simulink model "robosimulador"  (R2021b)
settings: Solver=VariableStepAuto  StartTime=0.0  StopTime=Time(length(Time))  MaxStep=1e-3  RelTol=1e-3
model workspace: external: MATLAB File /home/fabio/Desktop/Larc 2021/robosimulador_DataFile.m (data not in the file)
values from neighbouring files (symbols this model uses):
  j = length(Q)    [Cinematica_Comb.m]    (also in Cinematica_Heli_Coronal.m; Cinematica_Heli_Direta_Coronal.m; Cinematica_Heli_Sagital.m)
  Q = Qr    [Cinematica_Comb.m]
  X = zeros(1,14)    [Cinematica_Comb.m]    (also in Cinematica_Heli_Coronal.m = zeros(1,6); Cinematica_Heli_Direta_Coronal.m = zeros(1,6); Cinematica_Heli_Sagital.m = zeros(1,8))
  Y = zeros(1,14)    [Cinematica_Comb.m]    (also in Cinematica_Heli_Coronal.m = zeros(1,6); Cinematica_Heli_Direta_Coronal.m = zeros(1,6); Cinematica_Heli_Sagital.m = zeros(1,8))
  Z = zeros(1,14)    [Cinematica_Comb.m]    (also in Cinematica_Heli_Coronal.m = zeros(1,6); Cinematica_Heli_Direta_Coronal.m = zeros(1,6); Cinematica_Heli_Sagital.m = zeros(1,8))
undefined symbols (not defined in the file or in its folder): g, height_plane, plane_x, smiData, Time, Tmax, zzmp
libraries: nesl_utility x168, sm_lib x117, simulink x38, sharedutil x19, Contact_Forces_Lib x8
(part 6 of 6)

== system robosimulador/Robô/Lado Direito/Centro de Massa/ZMP Quadril/IW bat ==
  Constant1 : Constant  Value=smiData.Solid(10).PoI
  Constant4 : Constant  Value=smiData.Solid(10).MoI
  Demux1 : Demux  Outputs=3
  Demux2 : Demux  Outputs=3
  Gain : Gain  Gain=10e-6
  MATLAB Function1 : MATLAB Function  TreatAsAtomicUnit=on
  Multiply : Product  Multiplication=Matrix(*)
  PS-Simulink Converter1 : nesl_utility/PS-Simulink Converter  PhysicalDomain=network_engine_domain  SubClassName=ps_output  LeftPortType=input  RightPortType=output  PseudoPeriodic=off  Frequencies=[]  Unit=rad  AffineConversion=off
      settings: SourceProductBaseCode=PW,SS
  PS-Simulink Converter7 : nesl_utility/PS-Simulink Converter  PhysicalDomain=network_engine_domain  SubClassName=ps_output  LeftPortType=input  RightPortType=output  PseudoPeriodic=off  Frequencies=[]  Unit=rad/s  AffineConversion=off
      settings: SourceProductBaseCode=PW,SS
  PS-Simulink Converter8 : nesl_utility/PS-Simulink Converter  PhysicalDomain=network_engine_domain  SubClassName=ps_output  LeftPortType=input  RightPortType=output  PseudoPeriodic=off  Frequencies=[]  Unit=rad/s  AffineConversion=off
      settings: SourceProductBaseCode=PW,SS
  PS-Simulink Converter9 : nesl_utility/PS-Simulink Converter  PhysicalDomain=network_engine_domain  SubClassName=ps_output  LeftPortType=input  RightPortType=output  PseudoPeriodic=off  Frequencies=[]  Unit=rad/s  AffineConversion=off
      settings: SourceProductBaseCode=PW,SS
  Vector Concatenate : Concatenate  NumInputs=3
  wx : PMIOPort  Side=Left
  wy : PMIOPort  Port=2  Side=Left
  wz : PMIOPort  Port=3  Side=Left
  R : PMIOPort  Port=4  Side=Left
  Iw : Outport  VectorParamsAs1DForOutWhenUnconnected=off
  wires:
  Demux2/1 -> MATLAB Function1/2(Ix)
  Demux2/3 -> MATLAB Function1/4(Iz)
  PS-Simulink Converter7/1 -> Vector Concatenate/1
  Demux1/1 -> MATLAB Function1/5(Px)
  Demux1/2 -> MATLAB Function1/6(Py)
  Constant1/1 -> Demux1/1
  PS-Simulink Converter8/1 -> Vector Concatenate/2
  Vector Concatenate/1 -> Multiply/2
  PS-Simulink Converter9/1 -> Vector Concatenate/3
  MATLAB Function1/1(Ir) -> Gain/1
  Multiply/1 -> Iw/1
  Demux2/2 -> MATLAB Function1/3(Iy)
  Demux1/3 -> MATLAB Function1/7(Pz)
  Gain/1 -> Multiply/1
  Constant4/1 -> Demux2/1
  PS-Simulink Converter1/1 -> MATLAB Function1/1(R)
  connections:
  PS-Simulink Converter9/LConn1 -- wz/RConn1
  wx/RConn1 -- PS-Simulink Converter7/LConn1
  wy/RConn1 -- PS-Simulink Converter8/LConn1
  PS-Simulink Converter1/LConn1 -- R/RConn1

== system robosimulador/Robô/Lado Direito/Centro de Massa/ZMP Quadril1/IW bat ==
  Constant1 : Constant  Value=smiData.Solid(2).PoI
  Constant4 : Constant  Value=smiData.Solid(2).MoI
  Demux1 : Demux  Outputs=3
  Demux2 : Demux  Outputs=3
  Gain : Gain  Gain=10e-6
  MATLAB Function1 : MATLAB Function  TreatAsAtomicUnit=on
  Multiply : Product  Multiplication=Matrix(*)
  PS-Simulink Converter1 : nesl_utility/PS-Simulink Converter  PhysicalDomain=network_engine_domain  SubClassName=ps_output  LeftPortType=input  RightPortType=output  PseudoPeriodic=off  Frequencies=[]  Unit=rad  AffineConversion=off
      settings: SourceProductBaseCode=PW,SS
  PS-Simulink Converter7 : nesl_utility/PS-Simulink Converter  PhysicalDomain=network_engine_domain  SubClassName=ps_output  LeftPortType=input  RightPortType=output  PseudoPeriodic=off  Frequencies=[]  Unit=rad/s  AffineConversion=off
      settings: SourceProductBaseCode=PW,SS
  PS-Simulink Converter8 : nesl_utility/PS-Simulink Converter  PhysicalDomain=network_engine_domain  SubClassName=ps_output  LeftPortType=input  RightPortType=output  PseudoPeriodic=off  Frequencies=[]  Unit=rad/s  AffineConversion=off
      settings: SourceProductBaseCode=PW,SS
  PS-Simulink Converter9 : nesl_utility/PS-Simulink Converter  PhysicalDomain=network_engine_domain  SubClassName=ps_output  LeftPortType=input  RightPortType=output  PseudoPeriodic=off  Frequencies=[]  Unit=rad/s  AffineConversion=off
      settings: SourceProductBaseCode=PW,SS
  Vector Concatenate : Concatenate  NumInputs=3
  wx : PMIOPort  Side=Left
  wy : PMIOPort  Port=2  Side=Left
  wz : PMIOPort  Port=3  Side=Left
  R : PMIOPort  Port=4  Side=Left
  Iw : Outport  VectorParamsAs1DForOutWhenUnconnected=off
  wires:
  PS-Simulink Converter1/1 -> MATLAB Function1/1(R)
  Constant4/1 -> Demux2/1
  Gain/1 -> Multiply/1
  Demux1/3 -> MATLAB Function1/7(Pz)
  Demux2/2 -> MATLAB Function1/3(Iy)
  Multiply/1 -> Iw/1
  MATLAB Function1/1(Ir) -> Gain/1
  PS-Simulink Converter9/1 -> Vector Concatenate/3
  Vector Concatenate/1 -> Multiply/2
  PS-Simulink Converter8/1 -> Vector Concatenate/2
  Constant1/1 -> Demux1/1
  Demux1/2 -> MATLAB Function1/6(Py)
  Demux1/1 -> MATLAB Function1/5(Px)
  PS-Simulink Converter7/1 -> Vector Concatenate/1
  Demux2/3 -> MATLAB Function1/4(Iz)
  Demux2/1 -> MATLAB Function1/2(Ix)
  connections:
  PS-Simulink Converter1/LConn1 -- R/RConn1
  wy/RConn1 -- PS-Simulink Converter8/LConn1
  wx/RConn1 -- PS-Simulink Converter7/LConn1
  PS-Simulink Converter9/LConn1 -- wz/RConn1

== system robosimulador/Robô/Lado Direito/Centro de Massa/ZMP canela/IW bat ==
  Constant1 : Constant  Value=smiData.Solid(6).PoI
  Constant4 : Constant  Value=smiData.Solid(6).MoI
  Demux1 : Demux  Outputs=3
  Demux2 : Demux  Outputs=3
  Gain : Gain  Gain=10e-6
  MATLAB Function1 : MATLAB Function  TreatAsAtomicUnit=on
  Multiply : Product  Multiplication=Matrix(*)
  PS-Simulink Converter1 : nesl_utility/PS-Simulink Converter  PhysicalDomain=network_engine_domain  SubClassName=ps_output  LeftPortType=input  RightPortType=output  PseudoPeriodic=off  Frequencies=[]  Unit=rad  AffineConversion=off
      settings: SourceProductBaseCode=PW,SS
  PS-Simulink Converter7 : nesl_utility/PS-Simulink Converter  PhysicalDomain=network_engine_domain  SubClassName=ps_output  LeftPortType=input  RightPortType=output  PseudoPeriodic=off  Frequencies=[]  Unit=rad/s  AffineConversion=off
      settings: SourceProductBaseCode=PW,SS
  PS-Simulink Converter8 : nesl_utility/PS-Simulink Converter  PhysicalDomain=network_engine_domain  SubClassName=ps_output  LeftPortType=input  RightPortType=output  PseudoPeriodic=off  Frequencies=[]  Unit=rad/s  AffineConversion=off
      settings: SourceProductBaseCode=PW,SS
  PS-Simulink Converter9 : nesl_utility/PS-Simulink Converter  PhysicalDomain=network_engine_domain  SubClassName=ps_output  LeftPortType=input  RightPortType=output  PseudoPeriodic=off  Frequencies=[]  Unit=rad/s  AffineConversion=off
      settings: SourceProductBaseCode=PW,SS
  Vector Concatenate : Concatenate  NumInputs=3
  wx : PMIOPort  Side=Left
  wy : PMIOPort  Port=2  Side=Left
  wz : PMIOPort  Port=3  Side=Left
  R : PMIOPort  Port=4  Side=Left
  Iw : Outport  VectorParamsAs1DForOutWhenUnconnected=off
  wires:
  PS-Simulink Converter1/1 -> MATLAB Function1/1(R)
  Constant4/1 -> Demux2/1
  Gain/1 -> Multiply/1
  Demux1/3 -> MATLAB Function1/7(Pz)
  Demux2/2 -> MATLAB Function1/3(Iy)
  Multiply/1 -> Iw/1
  MATLAB Function1/1(Ir) -> Gain/1
  PS-Simulink Converter9/1 -> Vector Concatenate/3
  Vector Concatenate/1 -> Multiply/2
  PS-Simulink Converter8/1 -> Vector Concatenate/2
  Constant1/1 -> Demux1/1
  Demux1/2 -> MATLAB Function1/6(Py)
  Demux1/1 -> MATLAB Function1/5(Px)
  PS-Simulink Converter7/1 -> Vector Concatenate/1
  Demux2/3 -> MATLAB Function1/4(Iz)
  Demux2/1 -> MATLAB Function1/2(Ix)
  connections:
  PS-Simulink Converter1/LConn1 -- R/RConn1
  wy/RConn1 -- PS-Simulink Converter8/LConn1
  wx/RConn1 -- PS-Simulink Converter7/LConn1
  PS-Simulink Converter9/LConn1 -- wz/RConn1

== system robosimulador/Robô/Lado Direito/Centro de Massa/ZMP coxa/IW bat ==
  Constant1 : Constant  Value=smiData.Solid(5).PoI
  Constant4 : Constant  Value=smiData.Solid(5).MoI
  Demux1 : Demux  Outputs=3
  Demux2 : Demux  Outputs=3
  Gain : Gain  Gain=10e-6
  MATLAB Function1 : MATLAB Function  TreatAsAtomicUnit=on
  Multiply : Product  Multiplication=Matrix(*)
  PS-Simulink Converter1 : nesl_utility/PS-Simulink Converter  PhysicalDomain=network_engine_domain  SubClassName=ps_output  LeftPortType=input  RightPortType=output  PseudoPeriodic=off  Frequencies=[]  Unit=rad  AffineConversion=off
      settings: SourceProductBaseCode=PW,SS
  PS-Simulink Converter7 : nesl_utility/PS-Simulink Converter  PhysicalDomain=network_engine_domain  SubClassName=ps_output  LeftPortType=input  RightPortType=output  PseudoPeriodic=off  Frequencies=[]  Unit=rad/s  AffineConversion=off
      settings: SourceProductBaseCode=PW,SS
  PS-Simulink Converter8 : nesl_utility/PS-Simulink Converter  PhysicalDomain=network_engine_domain  SubClassName=ps_output  LeftPortType=input  RightPortType=output  PseudoPeriodic=off  Frequencies=[]  Unit=rad/s  AffineConversion=off
      settings: SourceProductBaseCode=PW,SS
  PS-Simulink Converter9 : nesl_utility/PS-Simulink Converter  PhysicalDomain=network_engine_domain  SubClassName=ps_output  LeftPortType=input  RightPortType=output  PseudoPeriodic=off  Frequencies=[]  Unit=rad/s  AffineConversion=off
      settings: SourceProductBaseCode=PW,SS
  Vector Concatenate : Concatenate  NumInputs=3
  wx : PMIOPort  Side=Left
  wy : PMIOPort  Port=2  Side=Left
  wz : PMIOPort  Port=3  Side=Left
  R : PMIOPort  Port=4  Side=Left
  Iw : Outport  VectorParamsAs1DForOutWhenUnconnected=off
  wires:
  Demux2/1 -> MATLAB Function1/2(Ix)
  Demux2/3 -> MATLAB Function1/4(Iz)
  PS-Simulink Converter7/1 -> Vector Concatenate/1
  Demux1/1 -> MATLAB Function1/5(Px)
  Demux1/2 -> MATLAB Function1/6(Py)
  Constant1/1 -> Demux1/1
  PS-Simulink Converter8/1 -> Vector Concatenate/2
  Vector Concatenate/1 -> Multiply/2
  PS-Simulink Converter9/1 -> Vector Concatenate/3
  MATLAB Function1/1(Ir) -> Gain/1
  Multiply/1 -> Iw/1
  Demux2/2 -> MATLAB Function1/3(Iy)
  Demux1/3 -> MATLAB Function1/7(Pz)
  Gain/1 -> Multiply/1
  Constant4/1 -> Demux2/1
  PS-Simulink Converter1/1 -> MATLAB Function1/1(R)
  connections:
  PS-Simulink Converter9/LConn1 -- wz/RConn1
  wx/RConn1 -- PS-Simulink Converter7/LConn1
  wy/RConn1 -- PS-Simulink Converter8/LConn1
  PS-Simulink Converter1/LConn1 -- R/RConn1

== system robosimulador/Robô/Lado Esquerdo/Centro de Massa/ZMP Ante Braco1/IW bat ==
  Constant1 : Constant  Value=smiData.Solid(4).PoI
  Constant4 : Constant  Value=smiData.Solid(4).MoI
  Demux1 : Demux  Outputs=3
  Demux2 : Demux  Outputs=3
  Gain : Gain  Gain=10e-6
  MATLAB Function1 : MATLAB Function  TreatAsAtomicUnit=on
  Multiply : Product  Multiplication=Matrix(*)
  PS-Simulink Converter1 : nesl_utility/PS-Simulink Converter  PhysicalDomain=network_engine_domain  SubClassName=ps_output  LeftPortType=input  RightPortType=output  PseudoPeriodic=off  Frequencies=[]  Unit=rad  AffineConversion=off
      settings: SourceProductBaseCode=PW,SS
  PS-Simulink Converter7 : nesl_utility/PS-Simulink Converter  PhysicalDomain=network_engine_domain  SubClassName=ps_output  LeftPortType=input  RightPortType=output  PseudoPeriodic=off  Frequencies=[]  Unit=rad/s  AffineConversion=off
      settings: SourceProductBaseCode=PW,SS
  PS-Simulink Converter8 : nesl_utility/PS-Simulink Converter  PhysicalDomain=network_engine_domain  SubClassName=ps_output  LeftPortType=input  RightPortType=output  PseudoPeriodic=off  Frequencies=[]  Unit=rad/s  AffineConversion=off
      settings: SourceProductBaseCode=PW,SS
  PS-Simulink Converter9 : nesl_utility/PS-Simulink Converter  PhysicalDomain=network_engine_domain  SubClassName=ps_output  LeftPortType=input  RightPortType=output  PseudoPeriodic=off  Frequencies=[]  Unit=rad/s  AffineConversion=off
      settings: SourceProductBaseCode=PW,SS
  Vector Concatenate : Concatenate  NumInputs=3
  wx : PMIOPort  Side=Left
  wy : PMIOPort  Port=2  Side=Left
  wz : PMIOPort  Port=3  Side=Left
  R : PMIOPort  Port=4  Side=Left
  Iw : Outport  VectorParamsAs1DForOutWhenUnconnected=off
  wires:
  Demux2/1 -> MATLAB Function1/2(Ix)
  Demux2/3 -> MATLAB Function1/4(Iz)
  PS-Simulink Converter7/1 -> Vector Concatenate/1
  Demux1/1 -> MATLAB Function1/5(Px)
  Demux1/2 -> MATLAB Function1/6(Py)
  Constant1/1 -> Demux1/1
  PS-Simulink Converter8/1 -> Vector Concatenate/2
  Vector Concatenate/1 -> Multiply/2
  PS-Simulink Converter9/1 -> Vector Concatenate/3
  MATLAB Function1/1(Ir) -> Gain/1
  Multiply/1 -> Iw/1
  Demux2/2 -> MATLAB Function1/3(Iy)
  Demux1/3 -> MATLAB Function1/7(Pz)
  Gain/1 -> Multiply/1
  Constant4/1 -> Demux2/1
  PS-Simulink Converter1/1 -> MATLAB Function1/1(R)
  connections:
  PS-Simulink Converter9/LConn1 -- wz/RConn1
  wx/RConn1 -- PS-Simulink Converter7/LConn1
  wy/RConn1 -- PS-Simulink Converter8/LConn1
  PS-Simulink Converter1/LConn1 -- R/RConn1

== system robosimulador/Robô/Lado Esquerdo/Centro de Massa/ZMP Braco/IW bat ==
  Constant1 : Constant  Value=smiData.Solid(8).PoI
  Constant4 : Constant  Value=smiData.Solid(8).MoI
  Demux1 : Demux  Outputs=3
  Demux2 : Demux  Outputs=3
  Gain : Gain  Gain=10e-6
  MATLAB Function1 : MATLAB Function  TreatAsAtomicUnit=on
  Multiply : Product  Multiplication=Matrix(*)
  PS-Simulink Converter1 : nesl_utility/PS-Simulink Converter  PhysicalDomain=network_engine_domain  SubClassName=ps_output  LeftPortType=input  RightPortType=output  PseudoPeriodic=off  Frequencies=[]  Unit=rad  AffineConversion=off
      settings: SourceProductBaseCode=PW,SS
  PS-Simulink Converter7 : nesl_utility/PS-Simulink Converter  PhysicalDomain=network_engine_domain  SubClassName=ps_output  LeftPortType=input  RightPortType=output  PseudoPeriodic=off  Frequencies=[]  Unit=rad/s  AffineConversion=off
      settings: SourceProductBaseCode=PW,SS
  PS-Simulink Converter8 : nesl_utility/PS-Simulink Converter  PhysicalDomain=network_engine_domain  SubClassName=ps_output  LeftPortType=input  RightPortType=output  PseudoPeriodic=off  Frequencies=[]  Unit=rad/s  AffineConversion=off
      settings: SourceProductBaseCode=PW,SS
  PS-Simulink Converter9 : nesl_utility/PS-Simulink Converter  PhysicalDomain=network_engine_domain  SubClassName=ps_output  LeftPortType=input  RightPortType=output  PseudoPeriodic=off  Frequencies=[]  Unit=rad/s  AffineConversion=off
      settings: SourceProductBaseCode=PW,SS
  Vector Concatenate : Concatenate  NumInputs=3
  wx : PMIOPort  Side=Left
  wy : PMIOPort  Port=2  Side=Left
  wz : PMIOPort  Port=3  Side=Left
  R : PMIOPort  Port=4  Side=Left
  Iw : Outport  VectorParamsAs1DForOutWhenUnconnected=off
  wires:
  PS-Simulink Converter1/1 -> MATLAB Function1/1(R)
  Constant4/1 -> Demux2/1
  Gain/1 -> Multiply/1
  Demux1/3 -> MATLAB Function1/7(Pz)
  Demux2/2 -> MATLAB Function1/3(Iy)
  Multiply/1 -> Iw/1
  MATLAB Function1/1(Ir) -> Gain/1
  PS-Simulink Converter9/1 -> Vector Concatenate/3
  Vector Concatenate/1 -> Multiply/2
  PS-Simulink Converter8/1 -> Vector Concatenate/2
  Constant1/1 -> Demux1/1
  Demux1/2 -> MATLAB Function1/6(Py)
  Demux1/1 -> MATLAB Function1/5(Px)
  PS-Simulink Converter7/1 -> Vector Concatenate/1
  Demux2/3 -> MATLAB Function1/4(Iz)
  Demux2/1 -> MATLAB Function1/2(Ix)
  connections:
  PS-Simulink Converter1/LConn1 -- R/RConn1
  wy/RConn1 -- PS-Simulink Converter8/LConn1
  wx/RConn1 -- PS-Simulink Converter7/LConn1
  PS-Simulink Converter9/LConn1 -- wz/RConn1

== system robosimulador/Robô/Lado Esquerdo/Centro de Massa/ZMP Ombro/IW bat ==
  Constant1 : Constant  Value=smiData.Solid(1).PoI
  Constant4 : Constant  Value=smiData.Solid(1).MoI
  Demux1 : Demux  Outputs=3
  Demux2 : Demux  Outputs=3
  Gain : Gain  Gain=10e-6
  MATLAB Function1 : MATLAB Function  TreatAsAtomicUnit=on
  Multiply : Product  Multiplication=Matrix(*)
  PS-Simulink Converter1 : nesl_utility/PS-Simulink Converter  PhysicalDomain=network_engine_domain  SubClassName=ps_output  LeftPortType=input  RightPortType=output  PseudoPeriodic=off  Frequencies=[]  Unit=rad  AffineConversion=off
      settings: SourceProductBaseCode=PW,SS
  PS-Simulink Converter7 : nesl_utility/PS-Simulink Converter  PhysicalDomain=network_engine_domain  SubClassName=ps_output  LeftPortType=input  RightPortType=output  PseudoPeriodic=off  Frequencies=[]  Unit=rad/s  AffineConversion=off
      settings: SourceProductBaseCode=PW,SS
  PS-Simulink Converter8 : nesl_utility/PS-Simulink Converter  PhysicalDomain=network_engine_domain  SubClassName=ps_output  LeftPortType=input  RightPortType=output  PseudoPeriodic=off  Frequencies=[]  Unit=rad/s  AffineConversion=off
      settings: SourceProductBaseCode=PW,SS
  PS-Simulink Converter9 : nesl_utility/PS-Simulink Converter  PhysicalDomain=network_engine_domain  SubClassName=ps_output  LeftPortType=input  RightPortType=output  PseudoPeriodic=off  Frequencies=[]  Unit=rad/s  AffineConversion=off
      settings: SourceProductBaseCode=PW,SS
  Vector Concatenate : Concatenate  NumInputs=3
  wx : PMIOPort  Side=Left
  wy : PMIOPort  Port=2  Side=Left
  wz : PMIOPort  Port=3  Side=Left
  R : PMIOPort  Port=4  Side=Left
  Iw : Outport  VectorParamsAs1DForOutWhenUnconnected=off
  wires:
  PS-Simulink Converter1/1 -> MATLAB Function1/1(R)
  Constant4/1 -> Demux2/1
  Gain/1 -> Multiply/1
  Demux1/3 -> MATLAB Function1/7(Pz)
  Demux2/2 -> MATLAB Function1/3(Iy)
  Multiply/1 -> Iw/1
  MATLAB Function1/1(Ir) -> Gain/1
  PS-Simulink Converter9/1 -> Vector Concatenate/3
  Vector Concatenate/1 -> Multiply/2
  PS-Simulink Converter8/1 -> Vector Concatenate/2
  Constant1/1 -> Demux1/1
  Demux1/2 -> MATLAB Function1/6(Py)
  Demux1/1 -> MATLAB Function1/5(Px)
  PS-Simulink Converter7/1 -> Vector Concatenate/1
  Demux2/3 -> MATLAB Function1/4(Iz)
  Demux2/1 -> MATLAB Function1/2(Ix)
  connections:
  PS-Simulink Converter1/LConn1 -- R/RConn1
  wy/RConn1 -- PS-Simulink Converter8/LConn1
  wx/RConn1 -- PS-Simulink Converter7/LConn1
  PS-Simulink Converter9/LConn1 -- wz/RConn1

== system robosimulador/Robô/Lado Esquerdo/Centro de Massa/ZMP Pe/IW bat ==
  Constant1 : Constant  Value=smiData.Solid(9).PoI
  Constant4 : Constant  Value=smiData.Solid(9).MoI
  Demux1 : Demux  Outputs=3
  Demux2 : Demux  Outputs=3
  Gain : Gain  Gain=10e-6
  MATLAB Function1 : MATLAB Function  TreatAsAtomicUnit=on
  Multiply : Product  Multiplication=Matrix(*)
  PS-Simulink Converter1 : nesl_utility/PS-Simulink Converter  PhysicalDomain=network_engine_domain  SubClassName=ps_output  LeftPortType=input  RightPortType=output  PseudoPeriodic=off  Frequencies=[]  Unit=rad  AffineConversion=off
      settings: SourceProductBaseCode=PW,SS
  PS-Simulink Converter7 : nesl_utility/PS-Simulink Converter  PhysicalDomain=network_engine_domain  SubClassName=ps_output  LeftPortType=input  RightPortType=output  PseudoPeriodic=off  Frequencies=[]  Unit=rad/s  AffineConversion=off
      settings: SourceProductBaseCode=PW,SS
  PS-Simulink Converter8 : nesl_utility/PS-Simulink Converter  PhysicalDomain=network_engine_domain  SubClassName=ps_output  LeftPortType=input  RightPortType=output  PseudoPeriodic=off  Frequencies=[]  Unit=rad/s  AffineConversion=off
      settings: SourceProductBaseCode=PW,SS
  PS-Simulink Converter9 : nesl_utility/PS-Simulink Converter  PhysicalDomain=network_engine_domain  SubClassName=ps_output  LeftPortType=input  RightPortType=output  PseudoPeriodic=off  Frequencies=[]  Unit=rad/s  AffineConversion=off
      settings: SourceProductBaseCode=PW,SS
  Vector Concatenate : Concatenate  NumInputs=3
  wx : PMIOPort  Side=Left
  wy : PMIOPort  Port=2  Side=Left
  wz : PMIOPort  Port=3  Side=Left
  R : PMIOPort  Port=4  Side=Left
  Iw : Outport  VectorParamsAs1DForOutWhenUnconnected=off
  wires:
  Demux2/1 -> MATLAB Function1/2(Ix)
  Demux2/3 -> MATLAB Function1/4(Iz)
  PS-Simulink Converter7/1 -> Vector Concatenate/1
  Demux1/1 -> MATLAB Function1/5(Px)
  Demux1/2 -> MATLAB Function1/6(Py)
  Constant1/1 -> Demux1/1
  PS-Simulink Converter8/1 -> Vector Concatenate/2
  Vector Concatenate/1 -> Multiply/2
  PS-Simulink Converter9/1 -> Vector Concatenate/3
  MATLAB Function1/1(Ir) -> Gain/1
  Multiply/1 -> Iw/1
  Demux2/2 -> MATLAB Function1/3(Iy)
  Demux1/3 -> MATLAB Function1/7(Pz)
  Gain/1 -> Multiply/1
  Constant4/1 -> Demux2/1
  PS-Simulink Converter1/1 -> MATLAB Function1/1(R)
  connections:
  PS-Simulink Converter9/LConn1 -- wz/RConn1
  wx/RConn1 -- PS-Simulink Converter7/LConn1
  wy/RConn1 -- PS-Simulink Converter8/LConn1
  PS-Simulink Converter1/LConn1 -- R/RConn1

== system robosimulador/Robô/Lado Esquerdo/Centro de Massa/ZMP Quadril/IW bat ==
  Constant1 : Constant  Value=smiData.Solid(10).PoI
  Constant4 : Constant  Value=smiData.Solid(10).MoI
  Demux1 : Demux  Outputs=3
  Demux2 : Demux  Outputs=3
  Gain : Gain  Gain=10e-6
  MATLAB Function1 : MATLAB Function  TreatAsAtomicUnit=on
  Multiply : Product  Multiplication=Matrix(*)
  PS-Simulink Converter1 : nesl_utility/PS-Simulink Converter  PhysicalDomain=network_engine_domain  SubClassName=ps_output  LeftPortType=input  RightPortType=output  PseudoPeriodic=off  Frequencies=[]  Unit=rad  AffineConversion=off
      settings: SourceProductBaseCode=PW,SS
  PS-Simulink Converter7 : nesl_utility/PS-Simulink Converter  PhysicalDomain=network_engine_domain  SubClassName=ps_output  LeftPortType=input  RightPortType=output  PseudoPeriodic=off  Frequencies=[]  Unit=rad/s  AffineConversion=off
      settings: SourceProductBaseCode=PW,SS
  PS-Simulink Converter8 : nesl_utility/PS-Simulink Converter  PhysicalDomain=network_engine_domain  SubClassName=ps_output  LeftPortType=input  RightPortType=output  PseudoPeriodic=off  Frequencies=[]  Unit=rad/s  AffineConversion=off
      settings: SourceProductBaseCode=PW,SS
  PS-Simulink Converter9 : nesl_utility/PS-Simulink Converter  PhysicalDomain=network_engine_domain  SubClassName=ps_output  LeftPortType=input  RightPortType=output  PseudoPeriodic=off  Frequencies=[]  Unit=rad/s  AffineConversion=off
      settings: SourceProductBaseCode=PW,SS
  Vector Concatenate : Concatenate  NumInputs=3
  wx : PMIOPort  Side=Left
  wy : PMIOPort  Port=2  Side=Left
  wz : PMIOPort  Port=3  Side=Left
  R : PMIOPort  Port=4  Side=Left
  Iw : Outport  VectorParamsAs1DForOutWhenUnconnected=off
  wires:
  Demux2/1 -> MATLAB Function1/2(Ix)
  Demux2/3 -> MATLAB Function1/4(Iz)
  PS-Simulink Converter7/1 -> Vector Concatenate/1
  Demux1/1 -> MATLAB Function1/5(Px)
  Demux1/2 -> MATLAB Function1/6(Py)
  Constant1/1 -> Demux1/1
  PS-Simulink Converter8/1 -> Vector Concatenate/2
  Vector Concatenate/1 -> Multiply/2
  PS-Simulink Converter9/1 -> Vector Concatenate/3
  MATLAB Function1/1(Ir) -> Gain/1
  Multiply/1 -> Iw/1
  Demux2/2 -> MATLAB Function1/3(Iy)
  Demux1/3 -> MATLAB Function1/7(Pz)
  Gain/1 -> Multiply/1
  Constant4/1 -> Demux2/1
  PS-Simulink Converter1/1 -> MATLAB Function1/1(R)
  connections:
  PS-Simulink Converter9/LConn1 -- wz/RConn1
  wx/RConn1 -- PS-Simulink Converter7/LConn1
  wy/RConn1 -- PS-Simulink Converter8/LConn1
  PS-Simulink Converter1/LConn1 -- R/RConn1

== system robosimulador/Robô/Lado Esquerdo/Centro de Massa/ZMP Quadril1/IW bat ==
  Constant1 : Constant  Value=smiData.Solid(2).PoI
  Constant4 : Constant  Value=smiData.Solid(2).MoI
  Demux1 : Demux  Outputs=3
  Demux2 : Demux  Outputs=3
  Gain : Gain  Gain=10e-6
  MATLAB Function1 : MATLAB Function  TreatAsAtomicUnit=on
  Multiply : Product  Multiplication=Matrix(*)
  PS-Simulink Converter1 : nesl_utility/PS-Simulink Converter  PhysicalDomain=network_engine_domain  SubClassName=ps_output  LeftPortType=input  RightPortType=output  PseudoPeriodic=off  Frequencies=[]  Unit=rad  AffineConversion=off
      settings: SourceProductBaseCode=PW,SS
  PS-Simulink Converter7 : nesl_utility/PS-Simulink Converter  PhysicalDomain=network_engine_domain  SubClassName=ps_output  LeftPortType=input  RightPortType=output  PseudoPeriodic=off  Frequencies=[]  Unit=rad/s  AffineConversion=off
      settings: SourceProductBaseCode=PW,SS
  PS-Simulink Converter8 : nesl_utility/PS-Simulink Converter  PhysicalDomain=network_engine_domain  SubClassName=ps_output  LeftPortType=input  RightPortType=output  PseudoPeriodic=off  Frequencies=[]  Unit=rad/s  AffineConversion=off
      settings: SourceProductBaseCode=PW,SS
  PS-Simulink Converter9 : nesl_utility/PS-Simulink Converter  PhysicalDomain=network_engine_domain  SubClassName=ps_output  LeftPortType=input  RightPortType=output  PseudoPeriodic=off  Frequencies=[]  Unit=rad/s  AffineConversion=off
      settings: SourceProductBaseCode=PW,SS
  Vector Concatenate : Concatenate  NumInputs=3
  wx : PMIOPort  Side=Left
  wy : PMIOPort  Port=2  Side=Left
  wz : PMIOPort  Port=3  Side=Left
  R : PMIOPort  Port=4  Side=Left
  Iw : Outport  VectorParamsAs1DForOutWhenUnconnected=off
  wires:
  PS-Simulink Converter1/1 -> MATLAB Function1/1(R)
  Constant4/1 -> Demux2/1
  Gain/1 -> Multiply/1
  Demux1/3 -> MATLAB Function1/7(Pz)
  Demux2/2 -> MATLAB Function1/3(Iy)
  Multiply/1 -> Iw/1
  MATLAB Function1/1(Ir) -> Gain/1
  PS-Simulink Converter9/1 -> Vector Concatenate/3
  Vector Concatenate/1 -> Multiply/2
  PS-Simulink Converter8/1 -> Vector Concatenate/2
  Constant1/1 -> Demux1/1
  Demux1/2 -> MATLAB Function1/6(Py)
  Demux1/1 -> MATLAB Function1/5(Px)
  PS-Simulink Converter7/1 -> Vector Concatenate/1
  Demux2/3 -> MATLAB Function1/4(Iz)
  Demux2/1 -> MATLAB Function1/2(Ix)
  connections:
  PS-Simulink Converter1/LConn1 -- R/RConn1
  wy/RConn1 -- PS-Simulink Converter8/LConn1
  wx/RConn1 -- PS-Simulink Converter7/LConn1
  PS-Simulink Converter9/LConn1 -- wz/RConn1

== system robosimulador/Robô/Lado Esquerdo/Centro de Massa/ZMP canela/IW bat ==
  Constant1 : Constant  Value=smiData.Solid(6).PoI
  Constant4 : Constant  Value=smiData.Solid(6).MoI
  Demux1 : Demux  Outputs=3
  Demux2 : Demux  Outputs=3
  Gain : Gain  Gain=10e-6
  MATLAB Function1 : MATLAB Function  TreatAsAtomicUnit=on
  Multiply : Product  Multiplication=Matrix(*)
  PS-Simulink Converter1 : nesl_utility/PS-Simulink Converter  PhysicalDomain=network_engine_domain  SubClassName=ps_output  LeftPortType=input  RightPortType=output  PseudoPeriodic=off  Frequencies=[]  Unit=rad  AffineConversion=off
      settings: SourceProductBaseCode=PW,SS
  PS-Simulink Converter7 : nesl_utility/PS-Simulink Converter  PhysicalDomain=network_engine_domain  SubClassName=ps_output  LeftPortType=input  RightPortType=output  PseudoPeriodic=off  Frequencies=[]  Unit=rad/s  AffineConversion=off
      settings: SourceProductBaseCode=PW,SS
  PS-Simulink Converter8 : nesl_utility/PS-Simulink Converter  PhysicalDomain=network_engine_domain  SubClassName=ps_output  LeftPortType=input  RightPortType=output  PseudoPeriodic=off  Frequencies=[]  Unit=rad/s  AffineConversion=off
      settings: SourceProductBaseCode=PW,SS
  PS-Simulink Converter9 : nesl_utility/PS-Simulink Converter  PhysicalDomain=network_engine_domain  SubClassName=ps_output  LeftPortType=input  RightPortType=output  PseudoPeriodic=off  Frequencies=[]  Unit=rad/s  AffineConversion=off
      settings: SourceProductBaseCode=PW,SS
  Vector Concatenate : Concatenate  NumInputs=3
  wx : PMIOPort  Side=Left
  wy : PMIOPort  Port=2  Side=Left
  wz : PMIOPort  Port=3  Side=Left
  R : PMIOPort  Port=4  Side=Left
  Iw : Outport  VectorParamsAs1DForOutWhenUnconnected=off
  wires:
  PS-Simulink Converter1/1 -> MATLAB Function1/1(R)
  Constant4/1 -> Demux2/1
  Gain/1 -> Multiply/1
  Demux1/3 -> MATLAB Function1/7(Pz)
  Demux2/2 -> MATLAB Function1/3(Iy)
  Multiply/1 -> Iw/1
  MATLAB Function1/1(Ir) -> Gain/1
  PS-Simulink Converter9/1 -> Vector Concatenate/3
  Vector Concatenate/1 -> Multiply/2
  PS-Simulink Converter8/1 -> Vector Concatenate/2
  Constant1/1 -> Demux1/1
  Demux1/2 -> MATLAB Function1/6(Py)
  Demux1/1 -> MATLAB Function1/5(Px)
  PS-Simulink Converter7/1 -> Vector Concatenate/1
  Demux2/3 -> MATLAB Function1/4(Iz)
  Demux2/1 -> MATLAB Function1/2(Ix)
  connections:
  PS-Simulink Converter1/LConn1 -- R/RConn1
  wy/RConn1 -- PS-Simulink Converter8/LConn1
  wx/RConn1 -- PS-Simulink Converter7/LConn1
  PS-Simulink Converter9/LConn1 -- wz/RConn1

== system robosimulador/Robô/Lado Esquerdo/Centro de Massa/ZMP coxa/IW bat ==
  Constant1 : Constant  Value=smiData.Solid(5).PoI
  Constant4 : Constant  Value=smiData.Solid(5).MoI
  Demux1 : Demux  Outputs=3
  Demux2 : Demux  Outputs=3
  Gain : Gain  Gain=10e-6
  MATLAB Function1 : MATLAB Function  TreatAsAtomicUnit=on
  Multiply : Product  Multiplication=Matrix(*)
  PS-Simulink Converter1 : nesl_utility/PS-Simulink Converter  PhysicalDomain=network_engine_domain  SubClassName=ps_output  LeftPortType=input  RightPortType=output  PseudoPeriodic=off  Frequencies=[]  Unit=rad  AffineConversion=off
      settings: SourceProductBaseCode=PW,SS
  PS-Simulink Converter7 : nesl_utility/PS-Simulink Converter  PhysicalDomain=network_engine_domain  SubClassName=ps_output  LeftPortType=input  RightPortType=output  PseudoPeriodic=off  Frequencies=[]  Unit=rad/s  AffineConversion=off
      settings: SourceProductBaseCode=PW,SS
  PS-Simulink Converter8 : nesl_utility/PS-Simulink Converter  PhysicalDomain=network_engine_domain  SubClassName=ps_output  LeftPortType=input  RightPortType=output  PseudoPeriodic=off  Frequencies=[]  Unit=rad/s  AffineConversion=off
      settings: SourceProductBaseCode=PW,SS
  PS-Simulink Converter9 : nesl_utility/PS-Simulink Converter  PhysicalDomain=network_engine_domain  SubClassName=ps_output  LeftPortType=input  RightPortType=output  PseudoPeriodic=off  Frequencies=[]  Unit=rad/s  AffineConversion=off
      settings: SourceProductBaseCode=PW,SS
  Vector Concatenate : Concatenate  NumInputs=3
  wx : PMIOPort  Side=Left
  wy : PMIOPort  Port=2  Side=Left
  wz : PMIOPort  Port=3  Side=Left
  R : PMIOPort  Port=4  Side=Left
  Iw : Outport  VectorParamsAs1DForOutWhenUnconnected=off
  wires:
  Demux2/1 -> MATLAB Function1/2(Ix)
  Demux2/3 -> MATLAB Function1/4(Iz)
  PS-Simulink Converter7/1 -> Vector Concatenate/1
  Demux1/1 -> MATLAB Function1/5(Px)
  Demux1/2 -> MATLAB Function1/6(Py)
  Constant1/1 -> Demux1/1
  PS-Simulink Converter8/1 -> Vector Concatenate/2
  Vector Concatenate/1 -> Multiply/2
  PS-Simulink Converter9/1 -> Vector Concatenate/3
  MATLAB Function1/1(Ir) -> Gain/1
  Multiply/1 -> Iw/1
  Demux2/2 -> MATLAB Function1/3(Iy)
  Demux1/3 -> MATLAB Function1/7(Pz)
  Gain/1 -> Multiply/1
  Constant4/1 -> Demux2/1
  PS-Simulink Converter1/1 -> MATLAB Function1/1(R)
  connections:
  PS-Simulink Converter9/LConn1 -- wz/RConn1
  wx/RConn1 -- PS-Simulink Converter7/LConn1
  wy/RConn1 -- PS-Simulink Converter8/LConn1
  PS-Simulink Converter1/LConn1 -- R/RConn1

== system robosimulador/Robô/Torso/CoM e ZMP Superior/ZMP Torso/IW bat ==
  Constant1 : Constant  Value=smiData.Solid(7).PoI
  Constant4 : Constant  Value=smiData.Solid(7).MoI
  Demux1 : Demux  Outputs=3
  Demux2 : Demux  Outputs=3
  Gain : Gain  Gain=10e-6
  MATLAB Function1 : MATLAB Function  TreatAsAtomicUnit=on
  Multiply : Product  Multiplication=Matrix(*)
  PS-Simulink Converter1 : nesl_utility/PS-Simulink Converter  PhysicalDomain=network_engine_domain  SubClassName=ps_output  LeftPortType=input  RightPortType=output  PseudoPeriodic=off  Frequencies=[]  Unit=rad  AffineConversion=off
      settings: SourceProductBaseCode=PW,SS
  PS-Simulink Converter7 : nesl_utility/PS-Simulink Converter  PhysicalDomain=network_engine_domain  SubClassName=ps_output  LeftPortType=input  RightPortType=output  PseudoPeriodic=off  Frequencies=[]  Unit=rad/s  AffineConversion=off
      settings: SourceProductBaseCode=PW,SS
  PS-Simulink Converter8 : nesl_utility/PS-Simulink Converter  PhysicalDomain=network_engine_domain  SubClassName=ps_output  LeftPortType=input  RightPortType=output  PseudoPeriodic=off  Frequencies=[]  Unit=rad/s  AffineConversion=off
      settings: SourceProductBaseCode=PW,SS
  PS-Simulink Converter9 : nesl_utility/PS-Simulink Converter  PhysicalDomain=network_engine_domain  SubClassName=ps_output  LeftPortType=input  RightPortType=output  PseudoPeriodic=off  Frequencies=[]  Unit=rad/s  AffineConversion=off
      settings: SourceProductBaseCode=PW,SS
  Vector Concatenate : Concatenate  NumInputs=3
  wx : PMIOPort  Side=Left
  wy : PMIOPort  Port=2  Side=Left
  wz : PMIOPort  Port=3  Side=Left
  R : PMIOPort  Port=4  Side=Left
  Iw : Outport  VectorParamsAs1DForOutWhenUnconnected=off
  wires:
  PS-Simulink Converter1/1 -> MATLAB Function1/1(R)
  Constant4/1 -> Demux2/1
  Gain/1 -> Multiply/1
  Demux1/3 -> MATLAB Function1/7(Pz)
  Demux2/2 -> MATLAB Function1/3(Iy)
  Multiply/1 -> Iw/1
  MATLAB Function1/1(Ir) -> Gain/1
  PS-Simulink Converter9/1 -> Vector Concatenate/3
  Vector Concatenate/1 -> Multiply/2
  PS-Simulink Converter8/1 -> Vector Concatenate/2
  Constant1/1 -> Demux1/1
  Demux1/2 -> MATLAB Function1/6(Py)
  Demux1/1 -> MATLAB Function1/5(Px)
  PS-Simulink Converter7/1 -> Vector Concatenate/1
  Demux2/3 -> MATLAB Function1/4(Iz)
  Demux2/1 -> MATLAB Function1/2(Ix)
  connections:
  PS-Simulink Converter1/LConn1 -- R/RConn1
  wy/RConn1 -- PS-Simulink Converter8/LConn1
  wx/RConn1 -- PS-Simulink Converter7/LConn1
  PS-Simulink Converter9/LConn1 -- wz/RConn1

== system robosimulador/Robô/Torso/CoM e ZMP Superior/ZMP cabeça /IW cab ==
  Constant1 : Constant  Value=smiData.Solid(3).PoI
  Constant4 : Constant  Value=smiData.Solid(3).MoI
  Demux1 : Demux  Outputs=3
  Demux2 : Demux  Outputs=3
  Gain : Gain  Gain=10e-6
  MATLAB Function1 : MATLAB Function  TreatAsAtomicUnit=on
  Multiply : Product  Multiplication=Matrix(*)
  PS-Simulink Converter1 : nesl_utility/PS-Simulink Converter  PhysicalDomain=network_engine_domain  SubClassName=ps_output  LeftPortType=input  RightPortType=output  PseudoPeriodic=off  Frequencies=[]  Unit=rad  AffineConversion=off
      settings: SourceProductBaseCode=PW,SS
  PS-Simulink Converter7 : nesl_utility/PS-Simulink Converter  PhysicalDomain=network_engine_domain  SubClassName=ps_output  LeftPortType=input  RightPortType=output  PseudoPeriodic=off  Frequencies=[]  Unit=rad/s  AffineConversion=off
      settings: SourceProductBaseCode=PW,SS
  PS-Simulink Converter8 : nesl_utility/PS-Simulink Converter  PhysicalDomain=network_engine_domain  SubClassName=ps_output  LeftPortType=input  RightPortType=output  PseudoPeriodic=off  Frequencies=[]  Unit=rad/s  AffineConversion=off
      settings: SourceProductBaseCode=PW,SS
  PS-Simulink Converter9 : nesl_utility/PS-Simulink Converter  PhysicalDomain=network_engine_domain  SubClassName=ps_output  LeftPortType=input  RightPortType=output  PseudoPeriodic=off  Frequencies=[]  Unit=rad/s  AffineConversion=off
      settings: SourceProductBaseCode=PW,SS
  Vector Concatenate : Concatenate  NumInputs=3
  wx : PMIOPort  Side=Left
  wy : PMIOPort  Port=2  Side=Left
  wz : PMIOPort  Port=3  Side=Left
  R : PMIOPort  Port=4  Side=Left
  Iw : Outport  VectorParamsAs1DForOutWhenUnconnected=off
  wires:
  Demux2/1 -> MATLAB Function1/2(Ix)
  Demux2/3 -> MATLAB Function1/4(Iz)
  PS-Simulink Converter7/1 -> Vector Concatenate/1
  Demux1/1 -> MATLAB Function1/5(Px)
  Demux1/2 -> MATLAB Function1/6(Py)
  Constant1/1 -> Demux1/1
  PS-Simulink Converter8/1 -> Vector Concatenate/2
  Vector Concatenate/1 -> Multiply/2
  PS-Simulink Converter9/1 -> Vector Concatenate/3
  MATLAB Function1/1(Ir) -> Gain/1
  Multiply/1 -> Iw/1
  Demux2/2 -> MATLAB Function1/3(Iy)
  Demux1/3 -> MATLAB Function1/7(Pz)
  Gain/1 -> Multiply/1
  Constant4/1 -> Demux2/1
  PS-Simulink Converter1/1 -> MATLAB Function1/1(R)
  connections:
  PS-Simulink Converter9/LConn1 -- wz/RConn1
  wx/RConn1 -- PS-Simulink Converter7/LConn1
  wy/RConn1 -- PS-Simulink Converter8/LConn1
  PS-Simulink Converter1/LConn1 -- R/RConn1

== system robosimulador/Robô/Torso/CoM e ZMP Superior/ZMP cabeça 1/IW cab ==
  Constant1 : Constant  Value=smiData.Solid(11).PoI
  Constant4 : Constant  Value=smiData.Solid(11).MoI
  Demux1 : Demux  Outputs=3
  Demux2 : Demux  Outputs=3
  Gain : Gain  Gain=10e-6
  MATLAB Function1 : MATLAB Function  TreatAsAtomicUnit=on
  Multiply : Product  Multiplication=Matrix(*)
  PS-Simulink Converter1 : nesl_utility/PS-Simulink Converter  PhysicalDomain=network_engine_domain  SubClassName=ps_output  LeftPortType=input  RightPortType=output  PseudoPeriodic=off  Frequencies=[]  Unit=rad  AffineConversion=off
      settings: SourceProductBaseCode=PW,SS
  PS-Simulink Converter7 : nesl_utility/PS-Simulink Converter  PhysicalDomain=network_engine_domain  SubClassName=ps_output  LeftPortType=input  RightPortType=output  PseudoPeriodic=off  Frequencies=[]  Unit=rad/s  AffineConversion=off
      settings: SourceProductBaseCode=PW,SS
  PS-Simulink Converter8 : nesl_utility/PS-Simulink Converter  PhysicalDomain=network_engine_domain  SubClassName=ps_output  LeftPortType=input  RightPortType=output  PseudoPeriodic=off  Frequencies=[]  Unit=rad/s  AffineConversion=off
      settings: SourceProductBaseCode=PW,SS
  PS-Simulink Converter9 : nesl_utility/PS-Simulink Converter  PhysicalDomain=network_engine_domain  SubClassName=ps_output  LeftPortType=input  RightPortType=output  PseudoPeriodic=off  Frequencies=[]  Unit=rad/s  AffineConversion=off
      settings: SourceProductBaseCode=PW,SS
  Vector Concatenate : Concatenate  NumInputs=3
  wx : PMIOPort  Side=Left
  wy : PMIOPort  Port=2  Side=Left
  wz : PMIOPort  Port=3  Side=Left
  R : PMIOPort  Port=4  Side=Left
  Iw : Outport  VectorParamsAs1DForOutWhenUnconnected=off
  wires:
  PS-Simulink Converter1/1 -> MATLAB Function1/1(R)
  Constant4/1 -> Demux2/1
  Gain/1 -> Multiply/1
  Demux1/3 -> MATLAB Function1/7(Pz)
  Demux2/2 -> MATLAB Function1/3(Iy)
  Multiply/1 -> Iw/1
  MATLAB Function1/1(Ir) -> Gain/1
  PS-Simulink Converter9/1 -> Vector Concatenate/3
  Vector Concatenate/1 -> Multiply/2
  PS-Simulink Converter8/1 -> Vector Concatenate/2
  Constant1/1 -> Demux1/1
  Demux1/2 -> MATLAB Function1/6(Py)
  Demux1/1 -> MATLAB Function1/5(Px)
  PS-Simulink Converter7/1 -> Vector Concatenate/1
  Demux2/3 -> MATLAB Function1/4(Iz)
  Demux2/1 -> MATLAB Function1/2(Ix)
  connections:
  PS-Simulink Converter1/LConn1 -- R/RConn1
  wy/RConn1 -- PS-Simulink Converter8/LConn1
  wx/RConn1 -- PS-Simulink Converter7/LConn1
  PS-Simulink Converter9/LConn1 -- wz/RConn1

== matlab function robosimulador/Robô/Lado Direito/Centro de Massa/ZMP canela/IW bat/MATLAB Function1 ==
  data: R input; Ir output; Ix input; Iy input; Iz input; Px input; Py input; Pz input
function Ir = fcn(R,Ix,Iy,Iz,Px,Py,Pz)
Ir=zeros(3,3);
I=[Ix Pz Py;Pz Iy Px;Py Px Iz];
Ir = R*I*transpose(R);

== matlab function robosimulador/Robô/Lado Direito/Centro de Massa/ZMP Pe/IW bat/MATLAB Function1 ==
  data: R input; Ir output; Ix input; Iy input; Iz input; Px input; Py input; Pz input
function Ir = fcn(R,Ix,Iy,Iz,Px,Py,Pz)
Ir=zeros(3,3);
I=[Ix Pz Py;Pz Iy Px;Py Px Iz];
Ir = R*I*transpose(R);

== matlab function robosimulador/Robô/Lado Esquerdo/Centro de Massa/ZMP Braco/IW bat/MATLAB Function1 ==
  data: R input; Ir output; Ix input; Iy input; Iz input; Px input; Py input; Pz input
function Ir = fcn(R,Ix,Iy,Iz,Px,Py,Pz)
Ir=zeros(3,3);
I=[Ix Pz Py;Pz Iy Px;Py Px Iz];
Ir = R*I*transpose(R);

== matlab function robosimulador/Robô/Lado Esquerdo/Centro de Massa/ZMP Ombro/IW bat/MATLAB Function1 ==
  data: R input; Ir output; Ix input; Iy input; Iz input; Px input; Py input; Pz input
function Ir = fcn(R,Ix,Iy,Iz,Px,Py,Pz)
Ir=zeros(3,3);
I=[Ix Pz Py;Pz Iy Px;Py Px Iz];
Ir = R*I*transpose(R);

== matlab function robosimulador/Robô/Lado Esquerdo/Centro de Massa/ZMP Pe/IW bat/MATLAB Function1 ==
  data: R input; Ir output; Ix input; Iy input; Iz input; Px input; Py input; Pz input
function Ir = fcn(R,Ix,Iy,Iz,Px,Py,Pz)
Ir=zeros(3,3);
I=[Ix Pz Py;Pz Iy Px;Py Px Iz];
Ir = R*I*transpose(R);

== matlab function robosimulador/Robô/Lado Direito/Centro de Massa/ZMP Quadril/IW bat/MATLAB Function1 ==
  data: R input; Ir output; Ix input; Iy input; Iz input; Px input; Py input; Pz input
function Ir = fcn(R,Ix,Iy,Iz,Px,Py,Pz)
Ir=zeros(3,3);
I=[Ix Pz Py;Pz Iy Px;Py Px Iz];
Ir = R*I*transpose(R);

== matlab function robosimulador/Robô/Lado Esquerdo/Centro de Massa/ZMP Quadril/IW bat/MATLAB Function1 ==
  data: R input; Ir output; Ix input; Iy input; Iz input; Px input; Py input; Pz input
function Ir = fcn(R,Ix,Iy,Iz,Px,Py,Pz)
Ir=zeros(3,3);
I=[Ix Pz Py;Pz Iy Px;Py Px Iz];
Ir = R*I*transpose(R);

== matlab function robosimulador/Robô/Lado Esquerdo/Centro de Massa/ZMP Quadril1/IW bat/MATLAB Function1 ==
  data: R input; Ir output; Ix input; Iy input; Iz input; Px input; Py input; Pz input
function Ir = fcn(R,Ix,Iy,Iz,Px,Py,Pz)
Ir=zeros(3,3);
I=[Ix Pz Py;Pz Iy Px;Py Px Iz];
Ir = R*I*transpose(R);

== matlab function robosimulador/Robô/Lado Esquerdo/Centro de Massa/ZMP canela/IW bat/MATLAB Function1 ==
  data: R input; Ir output; Ix input; Iy input; Iz input; Px input; Py input; Pz input
function Ir = fcn(R,Ix,Iy,Iz,Px,Py,Pz)
Ir=zeros(3,3);
I=[Ix Pz Py;Pz Iy Px;Py Px Iz];
Ir = R*I*transpose(R);

== matlab function robosimulador/Robô/Lado Esquerdo/Centro de Massa/ZMP coxa/IW bat/MATLAB Function1 ==
  data: R input; Ir output; Ix input; Iy input; Iz input; Px input; Py input; Pz input
function Ir = fcn(R,Ix,Iy,Iz,Px,Py,Pz)
Ir=zeros(3,3);
I=[Ix Pz Py;Pz Iy Px;Py Px Iz];
Ir = R*I*transpose(R);

== matlab function robosimulador/Robô/Torso/CoM e ZMP Superior/ZMP cabeça 1/IW cab/MATLAB Function1 ==
  data: R input; Ir output; Ix input; Iy input; Iz input; Px input; Py input; Pz input
function Ir = fcn(R,Ix,Iy,Iz,Px,Py,Pz)
Ir=zeros(3,3);
I=[Ix Pz Py;Pz Iy Px;Py Px Iz];
Ir = R*I*transpose(R);

== matlab function robosimulador/Robô/Torso/CoM e ZMP Superior/ZMP Torso/IW bat/MATLAB Function1 ==
  data: R input; Ir output; Ix input; Iy input; Iz input; Px input; Py input; Pz input
function Ir = fcn(R,Ix,Iy,Iz,Px,Py,Pz)
Ir=zeros(3,3);
I=[Ix Pz Py;Pz Iy Px;Py Px Iz];
Ir = R*I*transpose(R);

== matlab function robosimulador/Robô/Torso/CoM e ZMP Superior/ZMP cabeça /IW cab/MATLAB Function1 ==
  data: R input; Ir output; Ix input; Iy input; Iz input; Px input; Py input; Pz input
function Ir = fcn(R,Ix,Iy,Iz,Px,Py,Pz)
Ir=zeros(3,3);
I=[Ix Pz Py;Pz Iy Px;Py Px Iz];
Ir = R*I*transpose(R);

== matlab function robosimulador/Robô/Subsystem1/MATLAB Function ==
  data: Hxd input; xzmp output; yzmp output; Hyd input; Pxd input; Pyd input; Pzd input; Cmx input; Cmy input; mtot input; g input; zzmp input
function [xzmp,yzmp] = fcn(Hxd,Hyd,Pxd,Pyd,Pzd,Cmx,Cmy,mtot,g,zzmp)

xzmp=(mtot*g*Cmx+zzmp*Pxd-Hyd)/(mtot*g+Pzd);
yzmp=(mtot*g*Cmy+zzmp*Pyd+Hxd)/(mtot*g+Pzd);

== matlab function robosimulador/Robô/Lado Direito/Centro de Massa/ZMP Quadril1/IW bat/MATLAB Function1 ==
  data: R input; Ir output; Ix input; Iy input; Iz input; Px input; Py input; Pz input
function Ir = fcn(R,Ix,Iy,Iz,Px,Py,Pz)
Ir=zeros(3,3);
I=[Ix Pz Py;Pz Iy Px;Py Px Iz];
Ir = R*I*transpose(R);

== matlab function robosimulador/Robô/Lado Direito/Centro de Massa/ZMP Ombro/IW bat/MATLAB Function1 ==
  data: R input; Ir output; Ix input; Iy input; Iz input; Px input; Py input; Pz input
function Ir = fcn(R,Ix,Iy,Iz,Px,Py,Pz)
Ir=zeros(3,3);
I=[Ix Pz Py;Pz Iy Px;Py Px Iz];
Ir = R*I*transpose(R);

== matlab function robosimulador/Robô/Lado Esquerdo/Centro de Massa/ZMP Ante Braco1/IW bat/MATLAB Function1 ==
  data: R input; Ir output; Ix input; Iy input; Iz input; Px input; Py input; Pz input
function Ir = fcn(R,Ix,Iy,Iz,Px,Py,Pz)
Ir=zeros(3,3);
I=[Ix Pz Py;Pz Iy Px;Py Px Iz];
Ir = R*I*transpose(R);

== matlab function robosimulador/Robô/Lado Direito/Centro de Massa/ZMP Braco/IW bat/MATLAB Function1 ==
  data: R input; Ir output; Ix input; Iy input; Iz input; Px input; Py input; Pz input
function Ir = fcn(R,Ix,Iy,Iz,Px,Py,Pz)
Ir=zeros(3,3);
I=[Ix Pz Py;Pz Iy Px;Py Px Iz];
Ir = R*I*transpose(R);

== matlab function robosimulador/Robô/Lado Direito/Centro de Massa/ZMP Ante Braco1/IW bat/MATLAB Function1 ==
  data: R input; Ir output; Ix input; Iy input; Iz input; Px input; Py input; Pz input
function Ir = fcn(R,Ix,Iy,Iz,Px,Py,Pz)
Ir=zeros(3,3);
I=[Ix Pz Py;Pz Iy Px;Py Px Iz];
Ir = R*I*transpose(R);

== matlab function robosimulador/Robô/Lado Direito/Centro de Massa/ZMP coxa/IW bat/MATLAB Function1 ==
  data: R input; Ir output; Ix input; Iy input; Iz input; Px input; Py input; Pz input
function Ir = fcn(R,Ix,Iy,Iz,Px,Py,Pz)
Ir=zeros(3,3);
I=[Ix Pz Py;Pz Iy Px;Py Px Iz];
Ir = R*I*transpose(R);
